simulink model "satellite_final8"  (R2017b)
settings: Solver=FixedStepAuto  StartTime=0.0  StopTime=inf  FixedStep=0.002  RelTol=1e-3  EnableMultiTasking=on
libraries: dspmathops x14, simulink x2, WebSocketLibrary x1
settings Model: SimulationMode=external  Creator=tianlun  LastModifiedBy=tianlun
settings OptimizationCC: DefaultParameterBehavior=Inlined
settings DebuggingCC: ParameterTunabilityLossMsg=error
settings SFSimCC: MATLABDynamicMemAlloc=off
settings RTWCC: SystemTargetFile=ert_linux.tlc  MakeCommand=make_rtw OPTS=-DWITH_HW  TemplateMakefile=ert_linux.tmf  Description=Linux Embedded Coder  GenerateReport=on  IncludeHyperlinkInReport=on  LaunchReport=on  TargetLang=C++  GenerateTraceInfo=on  GenerateTraceReport=on  GenerateTraceReportSl=on  GenerateTraceReportSf=on  GenerateTraceReportEml=on
settings CodeAppCC: ForceParamTrailComments=on  IgnoreCustomStorageClasses=off  OperatorAnnotations=on  SimulinkDataObjDesc=on  SFDataObjDesc=on  InsertBlockDesc=on
settings STFCustomTargetCC: TargetLangStandard=C++03 (ISO)  MultiwordLength=256  ModelReferenceCompliant=off  CombineOutputUpdateFcns=on  ERTCustomFileBanners=on  SupportNonInlinedSFcns=off  RemoveResetFunc=on  SupportVariableSizeSignals=on  MATLABClassNameForMDSCustomization=Simulink.SoftwareTarget.ERTCustomization  GRTInterface=off  SystemTargetFile=ert_linux.tlc
settings ERTTargetCC: TargetLangStandard=C++03 (ISO)  ModelReferenceCompliant=off  ParMdlRefBuildCompliant=off  CompOptLevelCompliant=off  ConcurrentExecutionCompliant=off  SupportContinuousTime=on  SupportVariableSizeSignals=on  ModelStepFunctionPrototypeControlCompliant=off  CPPClassGenCompliant=off  UseToolchainInfoCompliant=off  ExtMode=on  InlinedParameterPlacement=NonHierarchical  ERTCustomFileTemplate=ert_linux_file_process.tlc

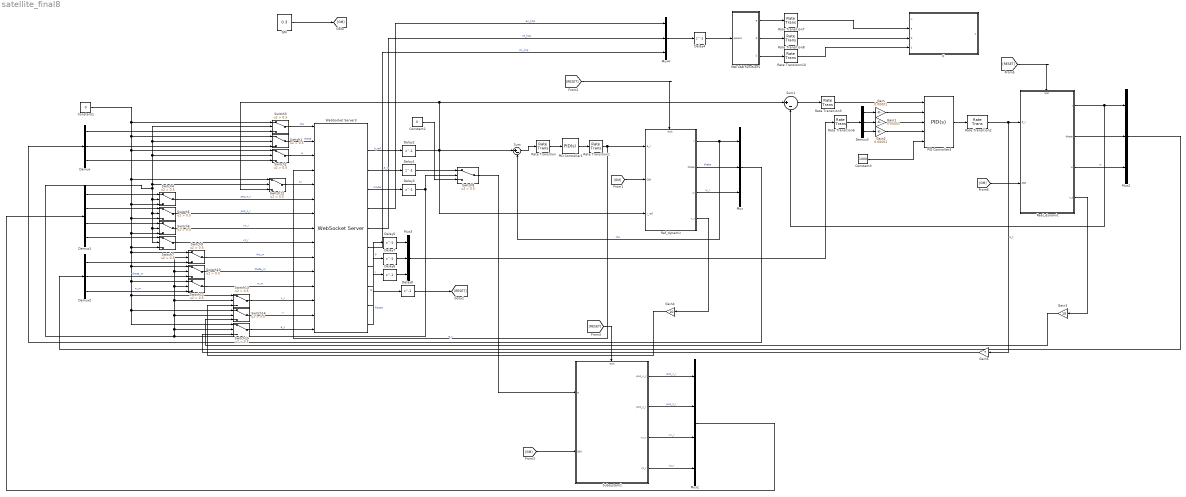
== system satellite_final8 ==
  Constant1 : Constant  Value=0
  Constant2 : Constant  Value=0
  Constant3 : Constant  Value=1000
  Delay{1,3,7..8} (4 alike) : Delay  DelayLength=1  InitialCondition=0
  Delay2 : Delay  DelayLength=1  InitialCondition=36
  Delay4 : Delay  DelayLength=1  InitialCondition=zeros(18,1)
  Delay5 : Delay  DelayLength=1  InitialCondition=1
  Delay6 : Delay  DelayLength=1  InitialCondition=1
  Demux : Demux  Outputs=3
  Demux1 : Demux
  Demux2 : Demux  Outputs=3
  Demux3 : Demux  Outputs=3
  GM : Constant  Value=0.3
  Gain : Gain  Gain=0.00001
  Gain1 : Gain  Gain=0.00001
  Gain2 : Gain  Gain=0.00001
  Gain3 : Gain  Gain=10
  Gain4 : Gain  Gain=10
  Gain5 : Gain  Gain=7
  K : Subsystem
  MATLAB Function5 : MATLAB Function  TreatAsAtomicUnit=on
  Mux{,2..4} (4 alike) : Mux  Inputs=3
  Mux1 : Mux
  PID Controller1 : simulink/Continuous/PID Controller  Controller=PID  TimeDomain=Continuous-time  SampleTime=-1  IntegratorMethod=Forward Euler  FilterMethod=Forward Euler  Form=Parallel  UseFilter=on  ControllerParametersSource=internal  P=0.00001  I=0  D=0.00001  N=1000  InitialConditionSource=internal  InitialConditionForIntegrator=0  InitialConditionForFilter=0  ExternalReset=none  LimitOutput=off  UpperSaturationLimit=inf  LowerSaturationLimit=-inf  LinearizeAsGain=on  AntiWindupMode=none  Kb=1  TrackingMode=off  Kt=1  PParamMin=[]  PParamMax=[]  IParamMin=[]  IParamMax=[]  DParamMin=[]  DParamMax=[]  NParamMin=[]  NParamMax=[]  KbParamMin=[]  KbParamMax=[]  KtParamMin=[]  KtParamMax=[]  POutMin=[]  POutMax=[]  IOutMin=[]  IOutMax=[]  DOutMin=[]  DOutMax=[]  NOutMin=[]  NOutMax=[]  KbOutMin=[]  KbOutMax=[]  KtOutMin=[]  KtOutMax=[]  IntegratorOutMin=[]  IntegratorOutMax=[]  FilterOutMin=[]  FilterOutMax=[]  SumOutMin=[]  SumOutMax=[]  SumI1OutMin=[]  SumI1OutMax=[]  SumI2OutMin=[]  SumI2OutMax=[]  SumI3OutMin=[]  SumI3OutMax=[]  SumDOutMin=[]  SumDOutMax=[]  SaturationOutMin=[]  SaturationOutMax=[]  IntegratorContinuousStateAttributes=''  IntegratorStateMustResolveToSignalObject=off  IntegratorRTWStateStorageClass=Auto  FilterContinuousStateAttributes=''  FilterStateMustResolveToSignalObject=off  FilterRTWStateStorageClass=Auto  DifferentiatorICPrevScaledInput=0  DifferentiatorOutMin=[]  DifferentiatorOutMax=[]  InitialConditionSetting=State (most efficient)  FilterDiffOutCoefMin=[]  FilterDiffOutCoefMax=[]  SumDenOutMin=[]  SumDenOutMax=[]  SumNumOutMin=[]  SumNumOutMax=[]  ReciprocalOutMin=[]  ReciprocalOutMax=[]  DivideOutMin=[]  DivideOutMax=[]  TunerSelectOption=Frequency Response Based
  PID Controller3 : simulink/Continuous/PID Controller  Controller=PID  TimeDomain=Continuous-time  SampleTime=-1  IntegratorMethod=Forward Euler  FilterMethod=Forward Euler  Form=Parallel  UseFilter=on  ControllerParametersSource=external  P=0.00001  I=0  D=0.00001  N=100  InitialConditionSource=internal  InitialConditionForIntegrator=0  InitialConditionForFilter=0  ExternalReset=none  LimitOutput=off  UpperSaturationLimit=inf  LowerSaturationLimit=-inf  LinearizeAsGain=on  AntiWindupMode=none  Kb=1  TrackingMode=off  Kt=1  PParamMin=[]  PParamMax=[]  IParamMin=[]  IParamMax=[]  DParamMin=[]  DParamMax=[]  NParamMin=[]  NParamMax=[]  KbParamMin=[]  KbParamMax=[]  KtParamMin=[]  KtParamMax=[]  POutMin=[]  POutMax=[]  IOutMin=[]  IOutMax=[]  DOutMin=[]  DOutMax=[]  NOutMin=[]  NOutMax=[]  KbOutMin=[]  KbOutMax=[]  KtOutMin=[]  KtOutMax=[]  IntegratorOutMin=[]  IntegratorOutMax=[]  FilterOutMin=[]  FilterOutMax=[]  SumOutMin=[]  SumOutMax=[]  SumI1OutMin=[]  SumI1OutMax=[]  SumI2OutMin=[]  SumI2OutMax=[]  SumI3OutMin=[]  SumI3OutMax=[]  SumDOutMin=[]  SumDOutMax=[]  SaturationOutMin=[]  SaturationOutMax=[]  IntegratorContinuousStateAttributes=''  IntegratorStateMustResolveToSignalObject=off  IntegratorRTWStateStorageClass=Auto  FilterContinuousStateAttributes=''  FilterStateMustResolveToSignalObject=off  FilterRTWStateStorageClass=Auto  DifferentiatorICPrevScaledInput=0  DifferentiatorOutMin=[]  DifferentiatorOutMax=[]  InitialConditionSetting=State (most efficient)  FilterDiffOutCoefMin=[]  FilterDiffOutCoefMax=[]  SumDenOutMin=[]  SumDenOutMax=[]  SumNumOutMin=[]  SumNumOutMax=[]  ReciprocalOutMin=[]  ReciprocalOutMax=[]  DivideOutMin=[]  DivideOutMax=[]  TunerSelectOption=Frequency Response Based
  Rate Transition{,1..3,6..8,10} (8 alike) : RateTransition
  Real_dynamic : Subsystem
  Ref_dynamic : Subsystem
  Subsystem1 : Subsystem
  Sum : Sum  Inputs=|+-
  Sum1 : Sum  Inputs=|+-
  Switch{1..15} (15 alike) : Switch  Criteria=u2 > Threshold  Threshold=0.5
  WebSocket Server3 : WebSocketLibrary/WebSocket Server  nOutputs=[1,1,1,6,6,6,1,1,1,1]  nInputs=[1,1,1,1,1,1,1,1,1,1,1,1,1,1,1]  splitInputs=[0,0,0,0,0,0,0,0,0,0,0,0,0,0,0]  jsonBlockConfig=''  totalSizeOut=7  totalSizeIn=7  nDiffInputs=6  address=localhost  port=30000  resource=/ws  sampleTime=0.04
  wires:
  Demux1/1 -> Switch4/1
  Demux1/3 -> Switch6/1
  Demux/3 -> Switch2/3
  Ref_dynamic/2(theta) -> Mux/2  "theta"
  Mux1/1 -> Demux1/1
  Sum/1 -> Rate Transition/1
  Delay1/1 -> Switch8/1
  [GM] -> Ref_dynamic/2(GM)
  Subsystem1/4(vz_r) -> Mux1/4  "vz_r"
  Ref_dynamic/3(w) -> Mux/3  "w_r"
  Demux/2 -> Switch1/3
  Demux1/4 -> Switch7/1
  [RESET] -> Real_dynamic/Reset
  Demux1/2 -> Switch5/1
  Demux/1 -> Switch3/3
  Constant2/1 -> Switch8/3
  Switch7/1 -> WebSocket Server3/9  "vz_r"
  Subsystem1/3(vx_r) -> Mux1/3  "vx_r"
  Delay2/1 -> Sum/1, Switch12/3, Sum1/1, Ref_dynamic/3(r_ref)
  Switch1/1 -> WebSocket Server3/2  "theta"
  Subsystem1/2(pos_z_r) -> Mux1/2  "pos_z_r"
  Subsystem1/1(pos_x_r) -> Mux1/1  "pos_x_r"
  Constant1/1 -> Switch15/1, Switch14/1, Switch13/1, Switch11/1, Switch10/1, Switch9/1, Switch7/3, Switch6/3, Switch5/3, Switch4/3, Switch12/1, Switch2/1, Switch1/1, Switch3/1
  Switch3/1 -> WebSocket Server3/1  "rho"
  Delay3/1 -> Switch8/2, Switch15/2, Switch14/2, Switch13/2, Switch11/2, Switch10/2, Switch9/2, Switch12/2, Switch3/2, Switch1/2, Switch2/2, Switch7/2, Switch6/2, Switch5/2, Switch4/2
  Mux/1 -> Demux/1
  GM/1 -> [GM]
  PID Controller1/1 -> Rate Transition1/1
  WebSocket Server3/3 -> Delay1/1  "a_t"
  Switch6/1 -> WebSocket Server3/8  "vx_r"
  WebSocket Server3/4 -> Delay3/1  "mode"
  Rate Transition/1 -> PID Controller1/1
  Rate Transition1/1 -> WebSocket Server3/4, Ref_dynamic/1(a_r)  "a_r"
  Ref_dynamic/1(r) -> Sum/2, Mux/1  "rho"
  [RESET] -> Subsystem1/Reset
  Switch8/1 -> Subsystem1/1(a)
  [RESET] -> Ref_dynamic/Reset
  WebSocket Server3/2 -> Delay2/1  "h_ref"
  [GM] -> Subsystem1/2(GM)
  Switch5/1 -> WebSocket Server3/7  "pos_z_r"
  Switch2/1 -> WebSocket Server3/3  "w"
  Switch4/1 -> WebSocket Server3/6  "pos_x_r"
  [GM] -> Real_dynamic/2(GM)
  Real_dynamic/3(w) -> Mux2/3  "w"
  Real_dynamic/2(theta) -> Mux2/2
  Sum1/1 -> Rate Transition3/1
  Rate Transition2/1 -> Gain5/1, Real_dynamic/1(a_r)  "a_t"
  Real_dynamic/1(r) -> Sum1/2, Mux2/1
  MATLAB Function5/2(b) -> Rate Transition8/1
  Mux4/1 -> Delay4/1
  MATLAB Function5/3(k) -> Rate Transition10/1
  MATLAB Function5/1(a) -> Rate Transition7/1
  Delay4/1 -> MATLAB Function5/1(param)
  WebSocket Server3/5 -> Mux4/1  "en_kzp"
  WebSocket Server3/6 -> Mux4/2  "re_kzp"
  WebSocket Server3/7 -> Mux4/3  "im_kzp"
  Rate Transition7/1 -> K/2(a)
  Rate Transition8/1 -> K/3(b)
  Rate Transition10/1 -> K/4(k)
  Mux2/1 -> Demux2/1
  Rate Transition3/1 -> PID Controller3/1
  PID Controller3/1 -> Rate Transition2/1
  WebSocket Server3/10 -> Delay6/1  "D"
  WebSocket Server3/9 -> Delay7/1  "I"
  WebSocket Server3/8 -> Delay5/1  "P"
  Delay5/1 -> Mux3/1
  Delay6/1 -> Mux3/3
  Delay7/1 -> Mux3/2
  Demux3/1 -> Gain/1
  Demux3/2 -> Gain1/1
  Demux3/3 -> Gain2/1
  Mux3/1 -> Rate Transition6/1
  Gain/1 -> PID Controller3/2
  Gain1/1 -> PID Controller3/3
  Constant3/1 -> PID Controller3/5
  Gain2/1 -> PID Controller3/4
  Rate Transition6/1 -> Demux3/1
  Switch9/1 -> WebSocket Server3/10  "rho_m"
  Demux2/1 -> Switch9/3
  Switch10/1 -> WebSocket Server3/11  "theta_m"
  Demux2/2 -> Switch10/3  "theta_m"
  Switch11/1 -> WebSocket Server3/12  "w_m"
  Demux2/3 -> Switch11/3  "w_m"
  WebSocket Server3/11 -> Delay8/1  "Reset"
  Delay8/1 -> [RESET]
  Switch12/1 -> WebSocket Server3/5  "hr"
  Switch13/1 -> WebSocket Server3/13  "v_r"
  Switch14/1 -> WebSocket Server3/14  "v"
  Switch15/1 -> WebSocket Server3/15  "a_t"
  Ref_dynamic/4(v_r) -> Gain4/1
  Real_dynamic/4(v_t) -> Gain3/1
  Gain4/1 -> Switch13/3
  Gain3/1 -> Switch14/3
  Gain5/1 -> Switch15/3

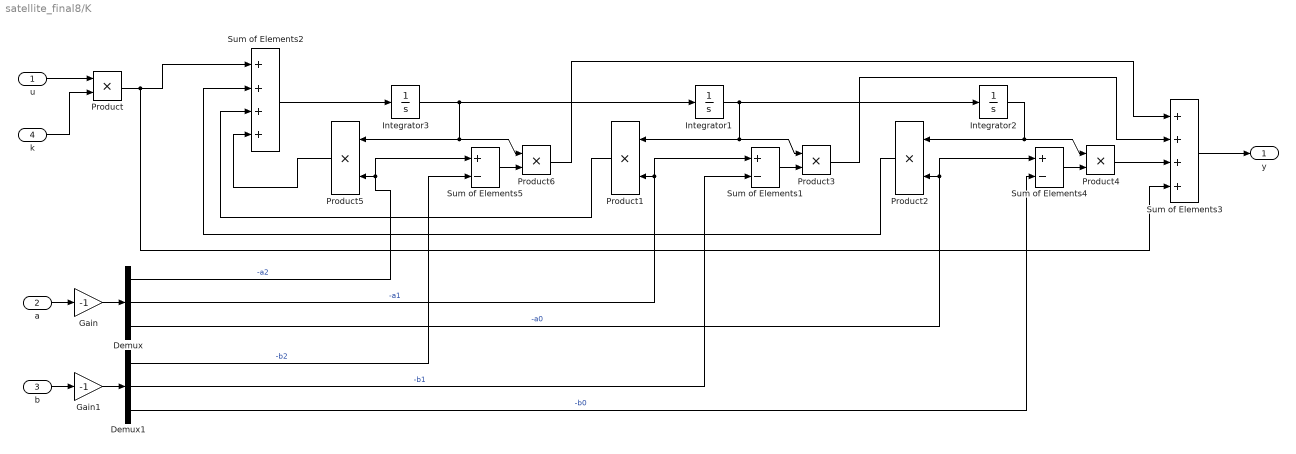
== system satellite_final8/K ==
  u : Inport
  a : Inport  Port=2
  b : Inport  Port=3
  k : Inport  Port=4
  Demux : Demux  Outputs=3
  Demux1 : Demux  Outputs=3
  Gain : Gain  Gain=-1
  Gain1 : Gain  Gain=-1
  Integrator1 : Integrator
  Integrator2 : Integrator
  Integrator3 : Integrator
  Product{,1..6} (7 alike) : Product
  Sum of Elements1 : Sum  Inputs=+-
  Sum of Elements2 : Sum  Inputs=++++
  Sum of Elements3 : Sum  Inputs=++++
  Sum of Elements4 : Sum  Inputs=+-
  Sum of Elements5 : Sum  Inputs=+-
  y : Outport
  wires:
  Product1/1 -> Sum of Elements2/3
  Product5/1 -> Sum of Elements2/4
  Integrator2/1 -> Product4/1, Product2/1
  Product4/1 -> Sum of Elements3/3
  Sum of Elements4/1 -> Product4/2
  Sum of Elements5/1 -> Product6/2
  Demux/1 -> Sum of Elements5/1, Product5/2  "-a2"
  Sum of Elements2/1 -> Integrator3/1
  u/1 -> Product/1
  Sum of Elements1/1 -> Product3/2
  Integrator3/1 -> Integrator1/1, Product6/1, Product5/1
  Product2/1 -> Sum of Elements2/2
  Product6/1 -> Sum of Elements3/1
  Demux1/2 -> Sum of Elements1/2  "-b1"
  Demux/2 -> Sum of Elements1/1, Product1/2  "-a1"
  Integrator1/1 -> Product3/1, Product1/1, Integrator2/1
  Demux/3 -> Sum of Elements4/1, Product2/2  "-a0"
  Demux1/3 -> Sum of Elements4/2  "-b0"
  Product3/1 -> Sum of Elements3/2
  Sum of Elements3/1 -> y/1
  a/1 -> Gain/1
  Gain/1 -> Demux/1
  b/1 -> Gain1/1
  Gain1/1 -> Demux1/1
  Demux1/1 -> Sum of Elements5/2  "-b2"
  Product/1 -> Sum of Elements3/4, Sum of Elements2/1
  k/1 -> Product/2

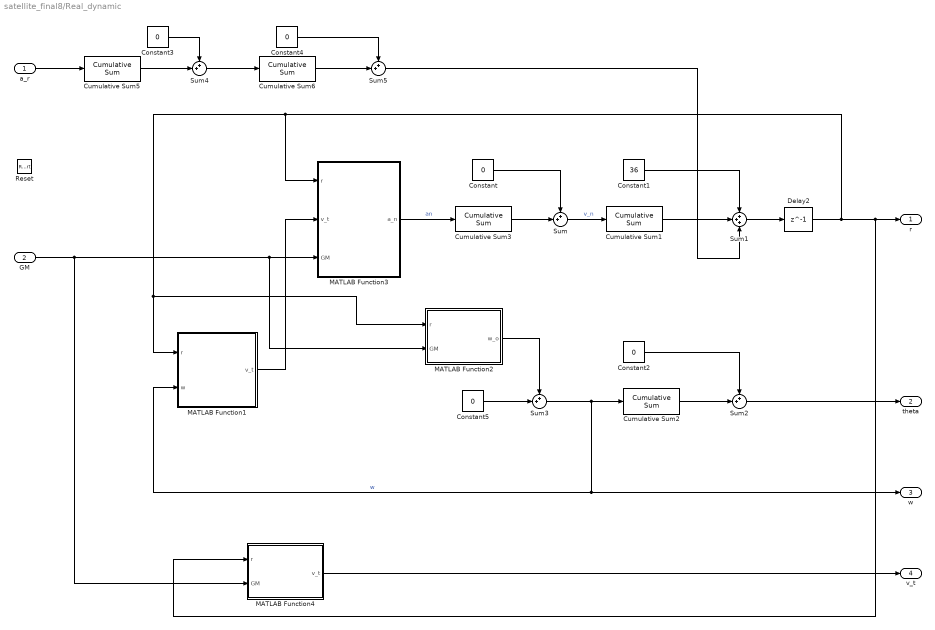
== system satellite_final8/Real_dynamic ==
  a_r : Inport
  GM : Inport  Port=2
  Reset : ResetPort  DisableCoverage=on  ResetTriggerType=either
  Constant{,2..5} (5 alike) : Constant  Value=0
  Constant1 : Constant  Value=36
  Cumulative Sum{1..3,5..6} (5 alike) : dspmathops/Cumulative Sum  dim=Channels (running sum)  InputProcessing=Columns as channels (frame based)  reset_popup=None  outputDataTypeStr=Inherit: Same as accumulator  outputLastDataTypeStr=Inherit: Same as accumulator  outputMin=[]  outputMax=[]  roundingMode=Floor  overflowMode=off
      settings: SourceProductName=DSP System Toolbox
  Delay2 : Delay  DelayLength=1  InitialCondition=36
  MATLAB Function1 : MATLAB Function  TreatAsAtomicUnit=on
  MATLAB Function2 : MATLAB Function  TreatAsAtomicUnit=on
  MATLAB Function3 : MATLAB Function  TreatAsAtomicUnit=on
  MATLAB Function4 : MATLAB Function  TreatAsAtomicUnit=on
  Sum{,2..5} (5 alike) : Sum  Inputs=++|
  Sum1 : Sum  Inputs=+++
  r : Outport
  theta : Outport  Port=2
  w : Outport  Port=3
  v_t : Outport  Port=4
  wires:
  MATLAB Function3/1(a_n) -> Cumulative Sum3/1  "an"
  Cumulative Sum3/1 -> Sum/2
  Sum/1 -> Cumulative Sum1/1  "v_n"
  Constant/1 -> Sum/1
  GM/1 -> MATLAB Function4/2(GM), MATLAB Function2/2(GM), MATLAB Function3/3(GM)
  Cumulative Sum1/1 -> Sum1/2
  Constant1/1 -> Sum1/1
  MATLAB Function1/1(v_t) -> MATLAB Function3/2(v_t)
  Sum3/1 -> w/1, MATLAB Function1/2(w), Cumulative Sum2/1  "w"
  Cumulative Sum2/1 -> Sum2/2
  Constant2/1 -> Sum2/1
  Sum2/1 -> theta/1
  MATLAB Function2/1(w_o) -> Sum3/1
  Constant5/1 -> Sum3/2
  Delay2/1 -> MATLAB Function2/1(r), MATLAB Function1/1(r), MATLAB Function3/1(r), MATLAB Function4/1(r), r/1
  Sum1/1 -> Delay2/1
  a_r/1 -> Cumulative Sum5/1
  Cumulative Sum5/1 -> Sum4/2
  Sum4/1 -> Cumulative Sum6/1
  Constant3/1 -> Sum4/1
  Cumulative Sum6/1 -> Sum5/2
  Constant4/1 -> Sum5/1
  Sum5/1 -> Sum1/3
  MATLAB Function4/1(v_t) -> v_t/1

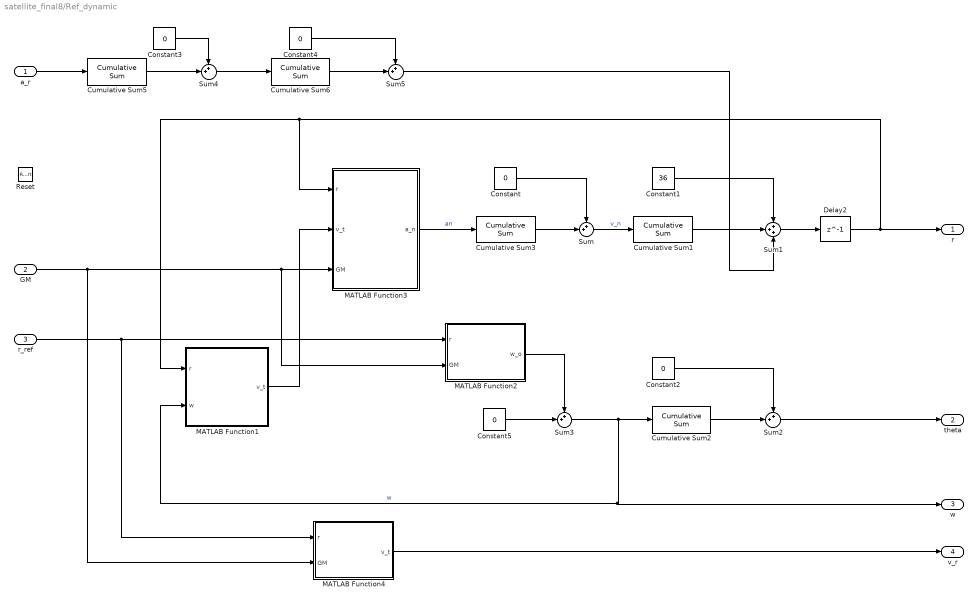
== system satellite_final8/Ref_dynamic ==
  a_r : Inport
  GM : Inport  Port=2
  r_ref : Inport  Port=3
  Reset : ResetPort  DisableCoverage=on  ResetTriggerType=either
  Constant{,2..5} (5 alike) : Constant  Value=0
  Constant1 : Constant  Value=36
  Cumulative Sum{1..3,5..6} (5 alike) : dspmathops/Cumulative Sum  dim=Channels (running sum)  InputProcessing=Columns as channels (frame based)  reset_popup=None  outputDataTypeStr=Inherit: Same as accumulator  outputLastDataTypeStr=Inherit: Same as accumulator  outputMin=[]  outputMax=[]  roundingMode=Floor  overflowMode=off
      settings: SourceProductName=DSP System Toolbox
  Delay2 : Delay  DelayLength=1  InitialCondition=36
  MATLAB Function1 : MATLAB Function  TreatAsAtomicUnit=on
  MATLAB Function2 : MATLAB Function  TreatAsAtomicUnit=on
  MATLAB Function3 : MATLAB Function  TreatAsAtomicUnit=on
  MATLAB Function4 : MATLAB Function  TreatAsAtomicUnit=on
  Sum{,2..5} (5 alike) : Sum  Inputs=++|
  Sum1 : Sum  Inputs=+++
  r : Outport
  theta : Outport  Port=2
  w : Outport  Port=3
  v_r : Outport  Port=4
  wires:
  MATLAB Function3/1(a_n) -> Cumulative Sum3/1  "an"
  Cumulative Sum3/1 -> Sum/2
  Sum/1 -> Cumulative Sum1/1  "v_n"
  Constant/1 -> Sum/1
  GM/1 -> MATLAB Function4/2(GM), MATLAB Function2/2(GM), MATLAB Function3/3(GM)
  Cumulative Sum1/1 -> Sum1/2
  Constant1/1 -> Sum1/1
  MATLAB Function1/1(v_t) -> MATLAB Function3/2(v_t)
  Sum3/1 -> w/1, MATLAB Function1/2(w), Cumulative Sum2/1  "w"
  Cumulative Sum2/1 -> Sum2/2
  Constant2/1 -> Sum2/1
  Sum2/1 -> theta/1
  MATLAB Function2/1(w_o) -> Sum3/1
  Constant5/1 -> Sum3/2
  Delay2/1 -> MATLAB Function1/1(r), MATLAB Function3/1(r), r/1
  Sum1/1 -> Delay2/1
  a_r/1 -> Cumulative Sum5/1
  Cumulative Sum5/1 -> Sum4/2
  Sum4/1 -> Cumulative Sum6/1
  Constant3/1 -> Sum4/1
  Cumulative Sum6/1 -> Sum5/2
  Constant4/1 -> Sum5/1
  Sum5/1 -> Sum1/3
  r_ref/1 -> MATLAB Function4/1(r), MATLAB Function2/1(r)
  MATLAB Function4/1(v_t) -> v_r/1

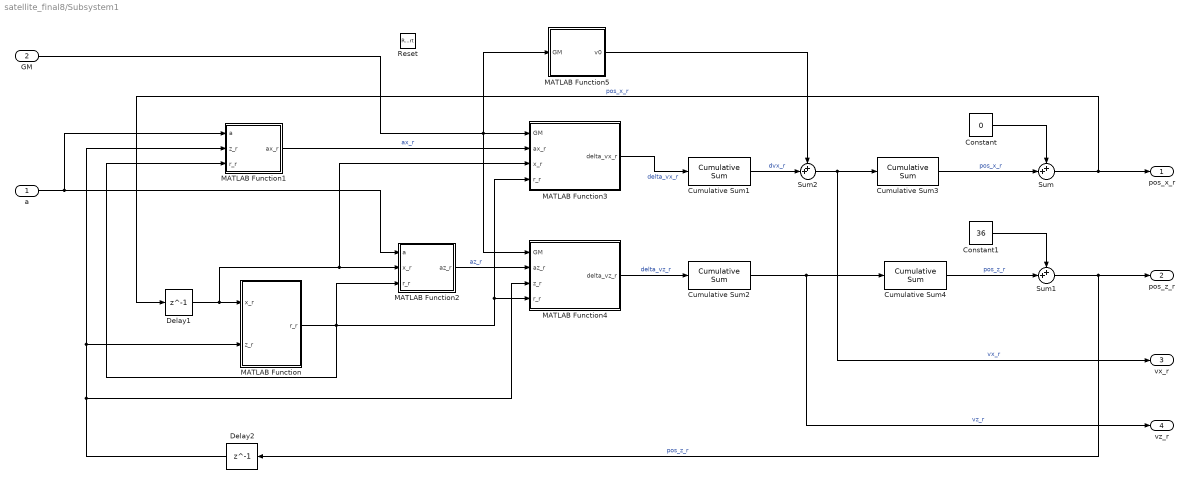
== system satellite_final8/Subsystem1 ==
  a : Inport
  GM : Inport  Port=2
  Reset : ResetPort  DisableCoverage=on  ResetTriggerType=either
  Constant : Constant  Value=0
  Constant1 : Constant  Value=36
  Cumulative Sum{1..4} (4 alike) : dspmathops/Cumulative Sum  dim=Channels (running sum)  InputProcessing=Columns as channels (frame based)  reset_popup=None  outputDataTypeStr=Inherit: Same as accumulator  outputLastDataTypeStr=Inherit: Same as accumulator  outputMin=[]  outputMax=[]  roundingMode=Floor  overflowMode=off
      settings: SourceProductName=DSP System Toolbox
  Delay1 : Delay  DelayLength=1  InitialCondition=0
  Delay2 : Delay  DelayLength=1  InitialCondition=36
  MATLAB Function : MATLAB Function  TreatAsAtomicUnit=on
  MATLAB Function1 : MATLAB Function  TreatAsAtomicUnit=on
  MATLAB Function2 : MATLAB Function  TreatAsAtomicUnit=on
  MATLAB Function3 : MATLAB Function  TreatAsAtomicUnit=on
  MATLAB Function4 : MATLAB Function  TreatAsAtomicUnit=on
  MATLAB Function5 : MATLAB Function  TreatAsAtomicUnit=on
  Sum : Sum  Inputs=++|
  Sum1 : Sum  Inputs=++|
  Sum2 : Sum  Inputs=++|
  pos_x_r : Outport
  pos_z_r : Outport  Port=2
  vx_r : Outport  Port=3
  vz_r : Outport  Port=4
  wires:
  Delay2/1 -> MATLAB Function1/2(z_r), MATLAB Function/2(z_r), MATLAB Function4/3(z_r)
  MATLAB Function2/1(az_r) -> MATLAB Function4/2(az_r)  "az_r"
  Sum2/1 -> vx_r/1, Cumulative Sum3/1  "vx_r"
  Constant/1 -> Sum/1
  Constant1/1 -> Sum1/1
  MATLAB Function3/1(delta_vx_r) -> Cumulative Sum1/1  "delta_vx_r"
  MATLAB Function5/1(v0) -> Sum2/1
  MATLAB Function/1(r_r) -> MATLAB Function3/4(r_r), MATLAB Function4/4(r_r), MATLAB Function1/3(r_r), MATLAB Function2/3(r_r)
  MATLAB Function1/1(ax_r) -> MATLAB Function3/2(ax_r)  "ax_r"
  MATLAB Function4/1(delta_vz_r) -> Cumulative Sum2/1  "delta_vz_r"
  Cumulative Sum1/1 -> Sum2/2  "dvx_r"
  Cumulative Sum2/1 -> vz_r/1, Cumulative Sum4/1  "vz_r"
  Cumulative Sum4/1 -> Sum1/2  "pos_z_r"
  Delay1/1 -> MATLAB Function3/3(x_r), MATLAB Function2/2(x_r), MATLAB Function/1(x_r)
  Cumulative Sum3/1 -> Sum/2  "pos_x_r"
  a/1 -> MATLAB Function1/1(a), MATLAB Function2/1(a)
  Sum/1 -> Delay1/1, pos_x_r/1  "pos_x_r"
  Sum1/1 -> Delay2/1, pos_z_r/1  "pos_z_r"
  GM/1 -> MATLAB Function3/1(GM), MATLAB Function5/1(GM), MATLAB Function4/1(GM)

== matlab function satellite_final8/Ref_dynamic/MATLAB Function4 ==
  data: r input; v_t output; GM input
function v_t = fcn(r,GM)

v_t = sqrt(GM/r);

== matlab function satellite_final8/Real_dynamic/MATLAB Function4 ==
  data: r input; v_t output; GM input
function v_t = fcn(r,GM)

v_t = sqrt(GM/r);

== matlab function satellite_final8/Real_dynamic/MATLAB Function1 ==
  data: r input; v_t output; w input
function v_t = fcn(r,w)

v_t = w*r;

== matlab function satellite_final8/Real_dynamic/MATLAB Function2 ==
  data: r input; w_o output; GM input
function w_o = fcn(r,GM)

w_o = sqrt(GM/36)/r;

== matlab function satellite_final8/Real_dynamic/MATLAB Function3 ==
  data: r input; a_n output; v_t input; GM input
function a_n = fcn(r,v_t,GM)

a_n = 0;

== matlab function satellite_final8/Ref_dynamic/MATLAB Function1 ==
  data: r input; v_t output; w input
function v_t = fcn(r,w)

v_t = w*r;

== matlab function satellite_final8/Ref_dynamic/MATLAB Function2 ==
  data: r input; w_o output; GM input
function w_o = fcn(r,GM)

w_o = sqrt(GM/36)/r;

== matlab function satellite_final8/Ref_dynamic/MATLAB Function3 ==
  data: r input; a_n output; v_t input; GM input
function a_n = fcn(r,v_t,GM)

a_n = 0;

== matlab function satellite_final8/Subsystem1/MATLAB Function ==
  data: x_r input; r_r output; z_r input
function r_r = fcn(x_r,z_r)
r_r=sqrt(x_r^2+z_r^2);

== matlab function satellite_final8/Subsystem1/MATLAB Function1 ==
  data: a input; ax_r output; z_r input; r_r input
function ax_r = fcn(a,z_r,r_r)
ax_r = a*z_r/r_r;

== matlab function satellite_final8/Subsystem1/MATLAB Function2 ==
  data: a input; az_r output; x_r input; r_r input
function az_r = fcn(a,x_r,r_r)
az_r=-a*x_r/r_r;

== matlab function satellite_final8/Subsystem1/MATLAB Function3 ==
  data: GM input; ax_r input; delta_vx_r output; x_r input; r_r input
function delta_vx_r = fcn(GM,ax_r,x_r,r_r)
delta_vx_r = ax_r-GM*x_r/r_r/r_r/r_r;

== matlab function satellite_final8/Subsystem1/MATLAB Function4 ==
  data: GM input; az_r input; delta_vz_r output; z_r input; r_r input
function delta_vz_r = fcn(GM,az_r,z_r,r_r)
delta_vz_r = az_r-GM*z_r/r_r/r_r/r_r;

== matlab function satellite_final8/Subsystem1/MATLAB Function5 ==
  data: GM input; v0 output
function v0 = fcn(GM)
v0=sqrt(GM/36);

== matlab function satellite_final8/MATLAB Function5 ==
  data: param input; a output; b output; k output
function [a,b,k] = tfcoeff(param)

u=param;
a=zeros(1,3);
b=zeros(1,3);
k=1;

persistent u_last
if isempty(u_last), u_last=zeros(18,1);end;

if 1 %u~=u_last
    u_last=u;
    
    % BUILD CHAR. POLYNOMIAL COMPONENTS
    z=[999i,999i,999i];
    kz=1;
    for i=1:3
        if u(i)==1
            z(i-0 ) = u(i+6 ) + u(i+12)*1i ;
        else
            z(i-0 ) = -100;
            kz = kz/100;
        end
    end
    zcoeff = poly(z);
    b=real(zcoeff(2:4));
    
    p=[999i,999i,999i];
    kp=1;
    for i=4:6
        if u(i)==1
            p(i-3 ) = u(i+6 ) + u(i+12)*1i ;
        else
            p(i-3 ) = -100;
            kp=kp/100;
        end
    end
    pcoeff = poly(p);
    a=real(pcoeff(2:4));
    
    k=kz/kp;
end
